simulink model "etc"  (R2024b)
settings: Solver=ode45  StartTime=0.0  StopTime=10.0  RelTol=1e-3  EnableMultiTasking=on
model workspace: external: MAT-File throttleData.mat (data not in the file)
undefined symbols (not defined in the file): Cs, digital_range, direction_range_analog, duty_range_analog, J, Kd, Ks, theta_eq, Ts, uint_range_10bit
settings Model: Creator=jrivitus  LastModifiedBy=student
settings SolverCC: MaxConsecutiveZCs=25  AlgebraicLoopSolver=TrustRegion
settings DataIOCC: LimitDataPoints=on  SaveFormat=Array  SaveOutput=off  SaveTime=off  ReturnWorkspaceOutputs=off
settings OptimizationCC: DefaultParameterBehavior=Inlined  ExpressionDepthLimit=2147483647  InitFltsAndDblsToZero=on  LifeSpan=1  EfficientTunableParamExpr=on
settings DebuggingCC: UnderspecifiedInitializationDetection=Classic  MergeDetectMultiDrivingBlocksExec=none  ParameterPrecisionLossMsg=none  FcnCallInpInsideContextMsg=warning  UnconnectedInputMsg=warning  UnconnectedOutputMsg=warning  UnconnectedLineMsg=warning  AllowSymbolicDim=off  StateNameClashWarn=warning  PregeneratedLibrarySubsystemCodeDiagnostic=none  SFUnexpectedBacktrackingDiag=warning  SFNoUnconditionalDefaultTransitionDiag=warning  SFExecutionAtInitializationDiag=none  ArithmeticOperatorsInVariantConditions=warning
settings HardwareCC: ProdLongLongMode=on
settings ModelReferenceCC: EnableRefExpFcnMdlSchedulingChecks=on  PropagateSignalLabelsOutOfModel=off
settings SFSimCC: SimUseLocalCustomCode=off  MATLABDynamicMemAlloc=off
settings RTWCC: Description=Embedded Coder  SystemTargetFile=ert.tlc  TemplateMakefile=ert_default_tmf  RTWUseLocalCustomCode=off  GPUComputeCapability=3.5  DLArmComputeVersion=19.05
settings CodeAppCC: IgnoreCustomStorageClasses=off  StateflowObjectComments=on
settings ERTTargetCC: MultiwordLength=2048  GenerateSampleERTMain=on  ERTCustomFileTemplate=example_file_process.tlc  ConvertIfToSwitch=off  SuppressUnreachableDefaultCases=off  DynamicArrayContainerType=coder::array
settings ConfigComp: CovSaveCumulativeToWorkspaceVar=on  CovExternalEMLEnable=off  CovSFcnEnable=off

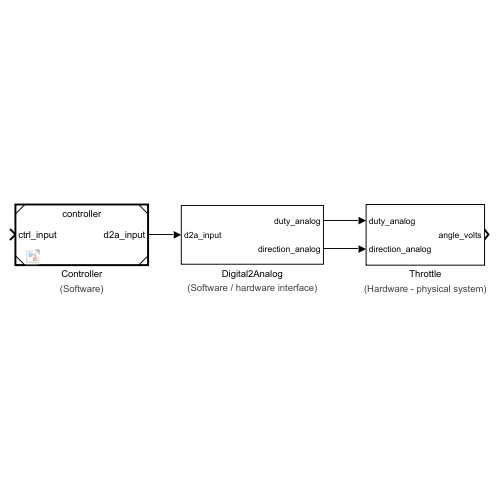
[thumbnail: Simulink's stored preview of the top-level diagram]
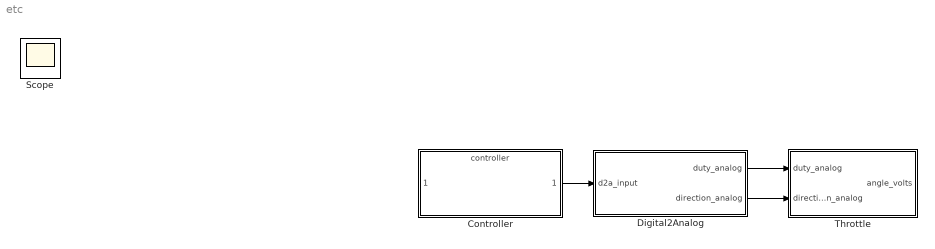
== system etc ==
  Controller : ModelReference  ModelNameDialog=controller  SimulationMode=Normal  ModelReferenceVersion=3.0
      settings: AttributesFormatString=(Software)
  Digital2Analog : Subsystem
      settings: AttributesFormatString=(Software / hardware interface)  MinAlgLoopOccurrences=on
  Throttle : Subsystem
      settings: AttributesFormatString=(Hardware - physical system)
  Scope : Scope
  wires:
  Controller/1 -> Digital2Analog/1(d2a_input)
  Digital2Analog/1(duty_analog) -> Throttle/1(duty_analog)
  Digital2Analog/2(direction_analog) -> Throttle/2(direction_analog)

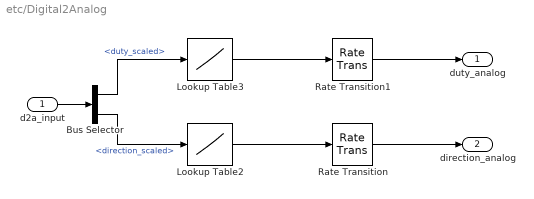
== system etc/Digital2Analog ==
  d2a_input : Inport  OutDataTypeStr=Bus: d2a_input_bus  PortDimensions=1  SampleTime=Ts
  Bus Selector : BusSelector  OutputSignals=duty_scaled,direction_scaled
  Lookup Table2 : Lookup_n-D  NumberOfTableDimensions=1  BreakpointsForDimension1=digital_range  Table=direction_range_analog  ExtrapMethod=Clip  OutDataTypeStr=double
      settings: AttributesFormatString=Output data type: %<OutDataTypeStr>
  Lookup Table3 : Lookup_n-D  NumberOfTableDimensions=1  BreakpointsForDimension1=uint_range_10bit  Table=duty_range_analog  ExtrapMethod=Clip  OutDataTypeStr=double
      settings: AttributesFormatString=Output data type: %<OutDataTypeStr>
  Rate Transition : RateTransition  Integrity=off  OutPortSampleTime=0
  Rate Transition1 : RateTransition  Integrity=off  OutPortSampleTime=0
  duty_analog : Outport  OutDataTypeStr=double  PortDimensions=1  SampleTime=0  VectorParamsAs1DForOutWhenUnconnected=off
  direction_analog : Outport  Port=2  OutDataTypeStr=double  PortDimensions=1  SampleTime=0  VectorParamsAs1DForOutWhenUnconnected=off
  wires:
  d2a_input/1 -> Bus Selector/1
  Lookup Table2/1 -> Rate Transition/1
  Lookup Table3/1 -> Rate Transition1/1
  Rate Transition1/1 -> duty_analog/1
  Rate Transition/1 -> direction_analog/1
  Bus Selector/1 -> Lookup Table3/1  "<duty_scaled>"
  Bus Selector/2 -> Lookup Table2/1  "<direction_scaled>"

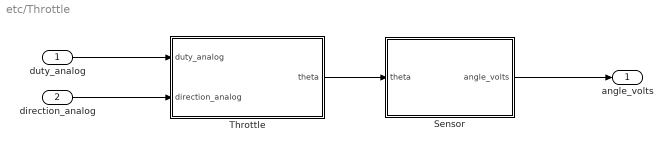
== system etc/Throttle ==
  duty_analog : Inport  OutDataTypeStr=double  PortDimensions=1  SampleTime=0
  direction_analog : Inport  Port=2  OutDataTypeStr=double  PortDimensions=1  SampleTime=0
  Sensor : Subsystem
  Throttle : Subsystem
  angle_volts : Outport  OutDataTypeStr=double  PortDimensions=1  SampleTime=0  VectorParamsAs1DForOutWhenUnconnected=off
  wires:
  duty_analog/1 -> Throttle/1(duty_analog)
  direction_analog/1 -> Throttle/2(direction_analog)
  Throttle/1(theta) -> Sensor/1(theta)
  Sensor/1(angle_volts) -> angle_volts/1

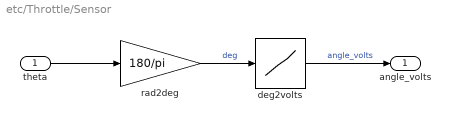
== system etc/Throttle/Sensor ==
  theta : Inport
  deg2volts : Lookup  InputValues=[0 90]  Table=[0.5 4.5]  LookUpMeth=Interpolation-Use End Values  SaturateOnIntegerOverflow=off
  rad2deg : Gain  Gain=180/pi  SaturateOnIntegerOverflow=on  OutDataTypeStr=Inherit: Same as input  ParamDataTypeStr=Inherit: Same as input
  angle_volts : Outport  VectorParamsAs1DForOutWhenUnconnected=off
  wires:
  theta/1 -> rad2deg/1
  deg2volts/1 -> angle_volts/1  "angle_volts"
  rad2deg/1 -> deg2volts/1  "deg"

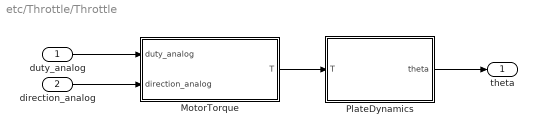
== system etc/Throttle/Throttle ==
  duty_analog : Inport
  direction_analog : Inport  Port=2
  MotorTorque : Subsystem
  PlateDynamics : Subsystem
  theta : Outport  VectorParamsAs1DForOutWhenUnconnected=off
  wires:
  MotorTorque/1(T) -> PlateDynamics/1(T)
  duty_analog/1 -> MotorTorque/1(duty_analog)
  direction_analog/1 -> MotorTorque/2(direction_analog)
  PlateDynamics/1(theta) -> theta/1

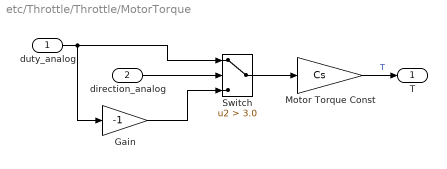
== system etc/Throttle/Throttle/MotorTorque ==
  duty_analog : Inport
  direction_analog : Inport  Port=2
  Gain : Gain  Gain=-1  SaturateOnIntegerOverflow=on  OutDataTypeStr=Inherit: Same as input  ParamDataTypeStr=Inherit: Same as input
  Motor Torque Const : Gain  Gain=Cs  SaturateOnIntegerOverflow=on  OutDataTypeStr=Inherit: Same as input  ParamDataTypeStr=Inherit: Same as input
  Switch : Switch  Criteria=u2 > Threshold  Threshold=3.0  SaturateOnIntegerOverflow=off  InputSameDT=off
  T : Outport  VectorParamsAs1DForOutWhenUnconnected=off
  wires:
  Switch/1 -> Motor Torque Const/1
  direction_analog/1 -> Switch/2
  duty_analog/1 -> Switch/1, Gain/1
  Gain/1 -> Switch/3
  Motor Torque Const/1 -> T/1  "T"

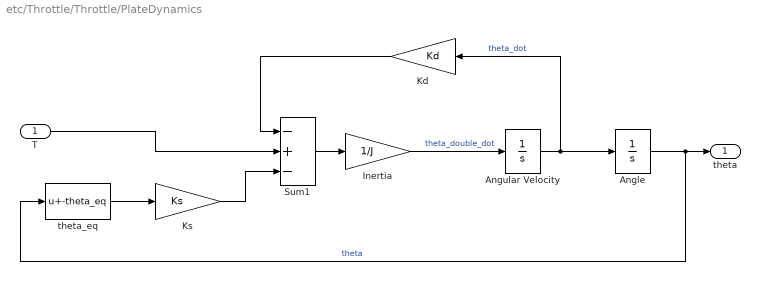
== system etc/Throttle/Throttle/PlateDynamics ==
  T : Inport
  Angle : Integrator  InitialCondition=theta_eq  LimitOutput=on  UpperSaturationLimit=pi/2  LowerSaturationLimit=0
      settings: AttributesFormatString=Initial condition: %<InitialCondition>\n%<LowerSaturationLimit> <= theta <= %<UpperSaturationLimit>
  Angular Velocity : Integrator
      settings: AttributesFormatString=Initial condition: %<InitialCondition>
  Inertia : Gain  Gain=1/J  SaturateOnIntegerOverflow=on  OutDataTypeStr=Inherit: Same as input  ParamDataTypeStr=Inherit: Same as input
  Kd : Gain  Gain=Kd  SaturateOnIntegerOverflow=on  OutDataTypeStr=Inherit: Same as input  ParamDataTypeStr=Inherit: Same as input
  Ks : Gain  Gain=Ks  SaturateOnIntegerOverflow=on  OutDataTypeStr=Inherit: Same as input  ParamDataTypeStr=Inherit: Same as input
  Sum1 : Sum  Inputs=-+-  SaturateOnIntegerOverflow=on
  theta_eq : Bias  Bias=-theta_eq  SaturateOnIntegerOverflow=off
  theta : Outport  VectorParamsAs1DForOutWhenUnconnected=off
  wires:
  theta_eq/1 -> Ks/1
  Angle/1 -> theta/1, theta_eq/1  "theta"
  Angular Velocity/1 -> Angle/1, Kd/1  "theta_dot"
  Inertia/1 -> Angular Velocity/1  "theta_double_dot"
  Sum1/1 -> Inertia/1
  Kd/1 -> Sum1/1
  Ks/1 -> Sum1/3
  T/1 -> Sum1/2
